simulink model "MotorDriverAveraged"  (R2026a)
settings: Solver=ode3  StopTime=5  FixedStep=0.0001
settings Model: Creator=drchi  LastModifiedBy=drchi

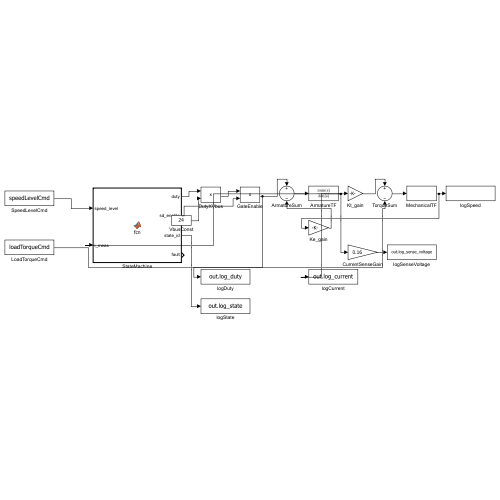
[thumbnail: Simulink's stored preview of the top-level diagram]
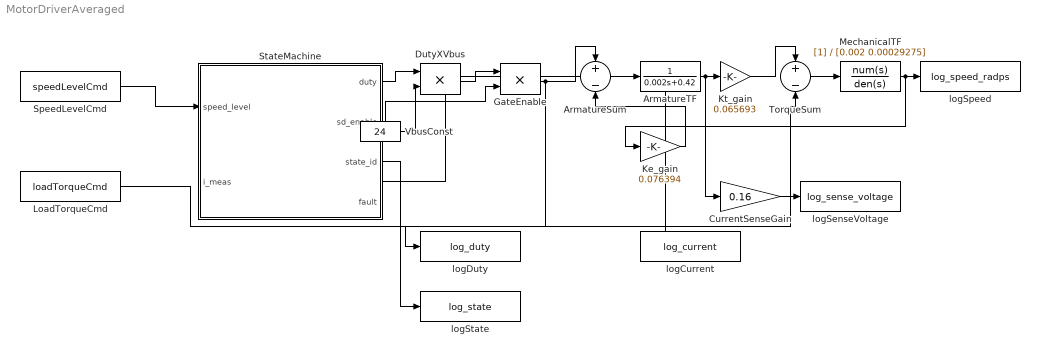
== system MotorDriverAveraged ==
  ArmatureSum : Sum  Inputs=+-
  ArmatureTF : TransferFcn  Denominator=[0.002 0.42]
  CurrentSenseGain : Gain  Gain=0.16
  DutyXVbus : Product
  GateEnable : Product
  Ke_gain : Gain  Gain=0.076394
  Kt_gain : Gain  Gain=0.065693
  LoadTorqueCmd : FromWorkspace  VariableName=loadTorqueCmd
  MechanicalTF : TransferFcn  Denominator=[0.002 0.00029275]
  SpeedLevelCmd : FromWorkspace  VariableName=speedLevelCmd
  StateMachine : MATLAB Function  TreatAsAtomicUnit=on
  TorqueSum : Sum  Inputs=+-
  VbusConst : Constant  Value=24
  logCurrent : ToWorkspace  VariableName=log_current  SaveFormat=Structure With Time  SampleTime=-1
  logDuty : ToWorkspace  VariableName=log_duty  SaveFormat=Structure With Time  SampleTime=-1
  logSenseVoltage : ToWorkspace  VariableName=log_sense_voltage  SaveFormat=Structure With Time  SampleTime=-1
  logSpeed : ToWorkspace  VariableName=log_speed_radps  SaveFormat=Structure With Time  SampleTime=-1
  logState : ToWorkspace  VariableName=log_state  SaveFormat=Structure With Time  SampleTime=-1
  wires:
  SpeedLevelCmd/1 -> StateMachine/1(speed_level)
  LoadTorqueCmd/1 -> TorqueSum/2
  StateMachine/1(duty) -> DutyXVbus/1
  VbusConst/1 -> DutyXVbus/2
  DutyXVbus/1 -> GateEnable/1
  StateMachine/2(sd_enable) -> GateEnable/2
  GateEnable/1 -> ArmatureSum/1, logDuty/1
  Ke_gain/1 -> ArmatureSum/2
  ArmatureSum/1 -> ArmatureTF/1
  ArmatureTF/1 -> Kt_gain/1, CurrentSenseGain/1, StateMachine/2(i_meas), logCurrent/1
  Kt_gain/1 -> TorqueSum/1
  TorqueSum/1 -> MechanicalTF/1
  MechanicalTF/1 -> Ke_gain/1, logSpeed/1
  StateMachine/3(state_id) -> logState/1
  CurrentSenseGain/1 -> logSenseVoltage/1

== matlab function MotorDriverAveraged/StateMachine ==
  settings: updateMethod=DISCRETE  sampleTime=0.0001
  data: speed_level input; duty output; i_meas input; sd_enable output; state_id output; fault output
function [duty, sd_enable, state_id, fault] = fcn(speed_level, i_meas)
%#codegen
% Ported from motor_driver_v2.ino state machine.
% state_id: 0=OFF 1=STARTING 2=RUNNING 3=BRAKING 4=FAULT
persistent state duty_val fault_timer ramp_step filtered_current
if isempty(state)
    state = 0; duty_val = 0; fault_timer = 0; ramp_step = 0; filtered_current = 0;
end

Ts = 1e-4;
DUTY_MAX = 0.95;
N_LEVELS = 10;
I_OVERCURRENT = 20;     % instantaneous trip, A
STALL_TIME = 1.0;       % s, sustained overcurrent -> stall fault
RAMP_STEP_PER_TICK = 0.002; % soft-start ramp rate (duty/tick) - TUNE THIS

target_duty = min(speed_level, N_LEVELS) / N_LEVELS * DUTY_MAX;

% --- replicate real ADC quantization + EMA filter from firmware ---
ADC_COUNTS_PER_AMP = (0.01 * 16) / (5/1024);  % shunt*gain / (Vref/1024)
i_adc_counts = round(i_meas * ADC_COUNTS_PER_AMP);
i_quantized = i_adc_counts / ADC_COUNTS_PER_AMP;
filtered_current = 0.1 * i_quantized + 0.9 * filtered_current;

% --- instantaneous overcurrent check (applies in any active state) ---
instant_oc = filtered_current > I_OVERCURRENT;

switch state
    case 0 % OFF
        duty_val = 0; fault_timer = 0;
        if speed_level > 0
            state = 1;
        end
    case 1 % STARTING (soft-start ramp toward target)
        if instant_oc
            fault_timer = fault_timer + Ts;
            if fault_timer >= STALL_TIME
                state = 4;
            end
        else
            fault_timer = 0;
        end
        if speed_level == 0
            state = 3; % BRAKING
        else
            duty_val = min(duty_val + RAMP_STEP_PER_TICK, target_duty);
            if duty_val >= target_duty - 1e-6
                state = 2;
            end
        end
    case 2 % RUNNING
        if instant_oc
            fault_timer = fault_timer + Ts;
            if fault_timer >= STALL_TIME
                state = 4; % stall fault
            end
        else
            fault_timer = 0;
        end
        if speed_level == 0
            state = 3;
        else
            duty_val = target_duty; % instant re-target on speed change
                                     % (matches firmware's per-press step,
                                     %  no re-ramp after initial start-up)
        end
    case 3 % BRAKING
        duty_val = 0;
        state = 0;
    case 4 % FAULT
        duty_val = 0;
        if speed_level == 0
            state = 0; fault_timer = 0; % fault clears on OFF command
        end
end

duty = round(duty_val * 799) / 799;
sd_enable = double(state ~= 4 && state ~= 0);
state_id = state;
fault = double(state == 4);
end
